simulink model "tanqueduplo"  (R2016a)
settings: Solver=VariableStepAuto  StartTime=0.0  StopTime=20  RelTol=1e-3
settings Model: Creator=Ítalo Renan  LastModifiedBy=Ítalo Renan

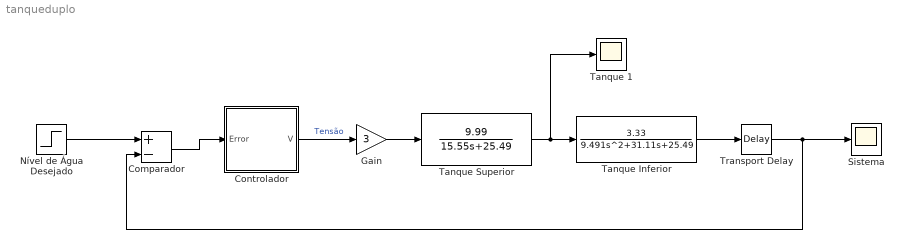
== system tanqueduplo ==
  Comparador : Sum  Inputs=+-
  Controlador : Subsystem
  Gain : Gain  Gain=3
  Nível de Água Desejado : Step  Time=0  After=15  SampleTime=0.01
  Sistema : Scope
  Tanque 1 : Scope
  Tanque Inferior : TransferFcn  Numerator=[3.33]  Denominator=[9.491 31.11 25.49]
  Tanque Superior : TransferFcn  Numerator=[9.99]  Denominator=[15.55 25.49]
  Transport Delay : TransportDelay
  wires:
  Controlador/1(V) -> Gain/1  "Tensão"
  Nível de Água Desejado/1 -> Comparador/1
  Comparador/1 -> Controlador/1(Error)
  Tanque Superior/1 -> Tanque 1/1, Tanque Inferior/1
  Transport Delay/1 -> Comparador/2, Sistema/1
  Gain/1 -> Tanque Superior/1
  Tanque Inferior/1 -> Transport Delay/1

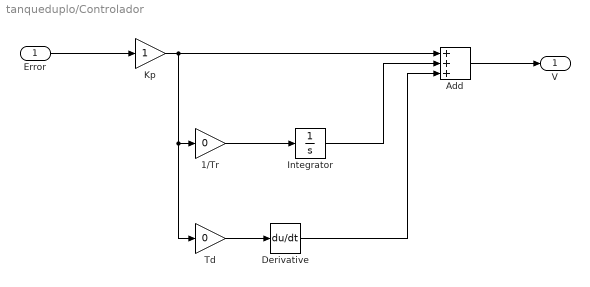
== system tanqueduplo/Controlador ==
  Error : Inport
  1/Tr : Gain  Gain=0
  Add : Sum  Inputs=+++
  Derivative : Derivative
  Integrator : Integrator  InitialCondition=0.
  Kp : Gain
  Td : Gain  Gain=0
  V : Outport
  wires:
  Error/1 -> Kp/1
  1/Tr/1 -> Integrator/1
  Td/1 -> Derivative/1
  Kp/1 -> Td/1, 1/Tr/1, Add/1
  Integrator/1 -> Add/2
  Derivative/1 -> Add/3
  Add/1 -> V/1
